simulink model "q6"  (R2023a)
settings: Solver=VariableStepAuto  StartTime=0.0  StopTime=10.0  RelTol=1e-3
settings Model: Creator=user  LastModifiedBy=user

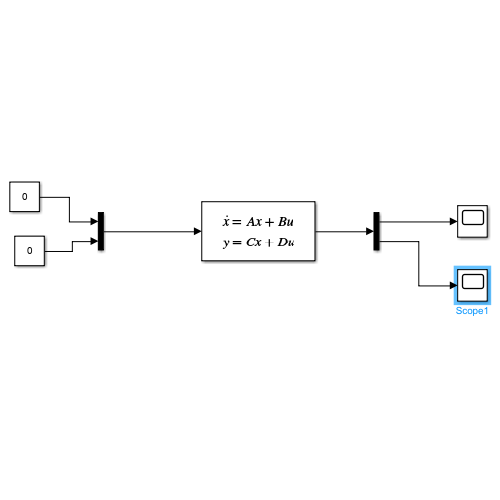
[thumbnail: Simulink's stored preview of the top-level diagram]
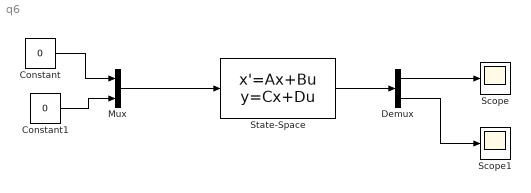
== system q6 ==
  Constant : Constant  Value=0
  Constant1 : Constant  Value=0
  Demux : Demux  Outputs=2
  Mux : Mux  Inputs=2
  Scope : Scope
  Scope1 : Scope
  State-Space : StateSpace  A=[0 1 0 0; 0 0 0 100; 0 0 0 1; 0 -100 0 0]  B=[0 0; 0 20; 0 0; 20 0]  C=[1 0 0 0; 0 0 1 0]  D=[0 0; 0 0]  InitialCondition=[1 0 pi/4 0]
  wires:
  Mux/1 -> State-Space/1
  State-Space/1 -> Demux/1
  Demux/1 -> Scope/1
  Demux/2 -> Scope1/1
  Constant1/1 -> Mux/2
  Constant/1 -> Mux/1
